simulink model "model"  (R2023b)
settings: Solver=VariableStepAuto  StartTime=0.0  StopTime=5  FixedStep=Tsi/10  RelTol=1e-4
undefined symbols (not defined in the file): B, B0, DiscIntNeverNeededParam, grtot, Hpp, Imax, In, Jm, Kdp_si, Ke, Ki_si, Kip_si, Kp_si, Kpp_si, Kppph_si, Kpppl_si, Kt, Kv, L, max_ppa_si, max_ppv_si, R, tauGp, Umax
libraries: simulink x10, slctrl_linear x1
(part 2 of 2)

== system model/EccB/current loop/current regulator ==
  current : Inport
  current_feedback : Inport  Port=2
  Scope : Scope  NumInputPorts=2
  Sum : Sum  Inputs=+-
  Sum2 : Sum
  Sum3 : Sum  Inputs=+-
  Sum4 : Sum  Inputs=++-
  Unit Delay : UnitDelay  SampleTime=-1  HasFrameUpgradeWarning=on
  integral gain : Gain  Gain=Ki_si*Tsi
  proportional gain : Gain  Gain=Kp_si
  voltage limitation : Saturate  UpperLimit=Umax  LowerLimit=-Umax
  voltage : Outport
  wires:
  voltage limitation/1 -> Scope/2, voltage/1, Sum3/2
  Sum3/1 -> Sum4/3
  Sum4/1 -> Unit Delay/1, Sum2/2  "ui(t)"
  Sum2/1 -> Sum3/1, Scope/1, voltage limitation/1  "u(t)"
  Sum/1 -> integral gain/1, proportional gain/1  "error"
  proportional gain/1 -> Sum2/1  "up(t)"
  current/1 -> Sum/1
  current_feedback/1 -> Sum/2
  Unit Delay/1 -> Sum4/1  "ui(t-1)"
  integral gain/1 -> Sum4/2

== system model/EccB/current loop/first order plant ==
  voltage : Inport
  Gain : Gain  Gain=1/tauM
  Gain5 : Gain  Gain=Kv
  Integrator : Integrator
  Integrator2 : Integrator
  Sum : Sum  Inputs=+-
  position : Outport
  velocity : Outport  Port=2
  wires:
  Integrator2/1 -> position/1
  voltage/1 -> Gain5/1
  Gain/1 -> Integrator/1
  Sum/1 -> Gain/1
  Integrator/1 -> Integrator2/1, velocity/1, Sum/2
  Gain5/1 -> Sum/1

== system model/EccB/current loop/power supply ==
  voltage setpoint : Inport
  Gain : Gain
  voltage : Outport
  wires:
  Gain/1 -> voltage/1
  voltage setpoint/1 -> Gain/1

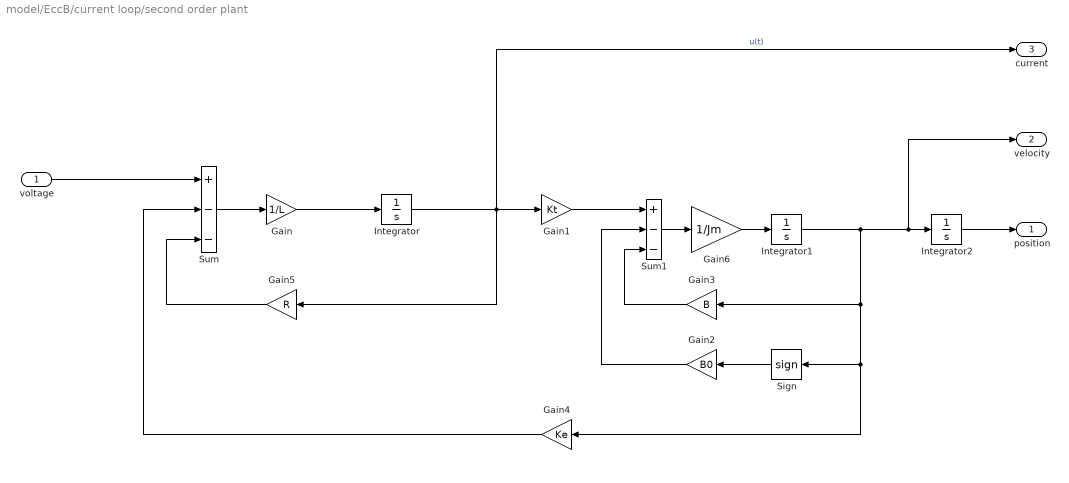
== system model/EccB/current loop/second order plant ==
  voltage : Inport
  Gain : Gain  Gain=1/L
  Gain1 : Gain  Gain=Kt
  Gain2 : Gain  Gain=B0
  Gain3 : Gain  Gain=B
  Gain4 : Gain  Gain=Ke
  Gain5 : Gain  Gain=R
  Gain6 : Gain  Gain=1/Jm
  Integrator : Integrator
  Integrator1 : Integrator
  Integrator2 : Integrator
  Sign : Signum
  Sum : Sum  Inputs=+--
  Sum1 : Sum  Inputs=+--
  position : Outport
  velocity : Outport  Port=2
  current : Outport  Port=3
  wires:
  Integrator2/1 -> position/1
  voltage/1 -> Sum/1
  Gain/1 -> Integrator/1
  Sum1/1 -> Gain6/1
  Gain5/1 -> Sum/3
  Gain6/1 -> Integrator1/1
  Gain4/1 -> Sum/2
  Sum/1 -> Gain/1
  Gain1/1 -> Sum1/1
  Sign/1 -> Gain2/1
  Gain3/1 -> Sum1/3
  Gain2/1 -> Sum1/2
  Integrator/1 -> current/1, Gain5/1, Gain1/1  "u(t)"
  Integrator1/1 -> velocity/1, Integrator2/1, Sign/1, Gain4/1, Gain3/1

== system model/EccB/path planner/devlta velocity ==
  Product : Product
  max acceleration : Constant  Value=max_ppa_si
  sampling time : Constant  Value=Tspp
  dw : Outport
  wires:
  sampling time/1 -> Product/1
  Product/1 -> dw/1
  max acceleration/1 -> Product/2

== system model/EccB/path planner/gain scheduler ==
  error : Inport
  Abs : Abs  SaturateOnIntegerOverflow=off
  Constant : Constant  Value=-Hpp
  Exp : Math
  Kp high : Constant  Value=Kppph_si
  Kp low : Constant  Value=Kpppl_si
  Product : Product
  Product1 : Product
  Sum : Sum  Inputs=+-
  Sum1 : Sum
  Km : Outport
  wires:
  Constant/1 -> Product/1
  Product/1 -> Exp/1
  Exp/1 -> Product1/1
  Abs/1 -> Product/2
  Kp low/1 -> Sum/1
  Kp high/1 -> Sum1/2, Sum/2
  Sum/1 -> Product1/2
  Product1/1 -> Sum1/1
  error/1 -> Abs/1
  Sum1/1 -> Km/1

== system model/EccB/path planner/setpoint correction ==
  speed : Inport
  feedback position : Inport  Port=2
  target position : Inport  Port=3
  AND : Logic  IconShape=distinctive  AllPortsSameDT=off  OutDataTypeStr=boolean
  AND1 : Logic  IconShape=distinctive  AllPortsSameDT=off  OutDataTypeStr=boolean
  Constant : Constant  Value=Active  OutDataTypeStr=boolean
  Constant2 : Constant  Value=0
  GreaterThan1 : RelationalOperator  Operator=>  OutDataTypeStr=boolean  RndMeth=Simplest  InputSameDT=off
  GreaterThan2 : RelationalOperator  Operator=<  OutDataTypeStr=boolean  RndMeth=Simplest  InputSameDT=off
  GreaterThan3 : RelationalOperator  Operator=<  OutDataTypeStr=boolean  RndMeth=Simplest  InputSameDT=off
  GreaterThan4 : RelationalOperator  Operator=>  OutDataTypeStr=boolean  RndMeth=Simplest  InputSameDT=off
  OR : Logic  Operator=OR  IconShape=distinctive  AllPortsSameDT=off  OutDataTypeStr=boolean
  Switch : Switch  Criteria=u2 > Threshold  SaturateOnIntegerOverflow=off  InputSameDT=off
  Terminator : Terminator
  motor velocity : Outport
  motor position : Outport  Port=2
  wires:
  GreaterThan3/1 -> AND1/1
  GreaterThan1/1 -> AND/2
  GreaterThan4/1 -> AND/1
  AND1/1 -> OR/2
  AND/1 -> OR/1
  Switch/1 -> motor position/1
  GreaterThan2/1 -> AND1/2
  speed/1 -> motor velocity/1  "filtered velocity"
  feedback position/1 -> GreaterThan2/2, Switch/1, GreaterThan1/2
  Constant2/1 -> GreaterThan3/2, GreaterThan4/2
  Constant/1 -> Switch/2
  OR/1 -> Terminator/1
  target position/1 -> Switch/3, GreaterThan3/1, GreaterThan2/1, GreaterThan1/1, GreaterThan4/1

== system model/EccB/position regulator/Integral + ant-windup ==
  error : Inport
  ui_old_sat : Inport  Port=2
  ui_old_no_sat : Inport  Port=3
  AND1 : Logic  IconShape=distinctive  AllPortsSameDT=off  OutDataTypeStr=boolean
  Constant1 : Constant  Value=0
  Ki : Gain  Gain=Kip_si*Tsp
  Relational Operator1 : RelationalOperator  Operator=~=  OutDataTypeStr=boolean  RndMeth=Simplest  InputSameDT=off
  Relational Operator3 : RelationalOperator  Operator=~=  OutDataTypeStr=boolean  RndMeth=Simplest  InputSameDT=off
  Sign1 : Signum
  Sign2 : Signum
  Sum1 : Sum
  Switch1 : Switch  Criteria=u2 > Threshold  SaturateOnIntegerOverflow=off  InputSameDT=off
  Unit Delay : UnitDelay  SampleTime=-1  HasFrameUpgradeWarning=on
  saturation : Saturate  UpperLimit=Imax  LowerLimit=-Imax
  ui (t) : Outport
  wires:
  Sign2/1 -> Relational Operator3/2
  error/1 -> Ki/1, Sign2/1
  Constant1/1 -> Switch1/1
  ui_old_sat/1 -> Relational Operator1/1
  ui_old_no_sat/1 -> Sign1/1, Relational Operator1/2
  Relational Operator3/1 -> AND1/2
  Relational Operator1/1 -> AND1/1
  Sign1/1 -> Relational Operator3/1
  AND1/1 -> Switch1/2
  Switch1/1 -> ui (t)/1, Unit Delay/1
  Sum1/1 -> saturation/1  "ui(t)"
  Ki/1 -> Sum1/1  "u(t)"
  Unit Delay/1 -> Sum1/2
  saturation/1 -> Switch1/3

== system model/LinB/current loop/current regulator ==
  current : Inport
  current_feedback : Inport  Port=2
  Scope : Scope  NumInputPorts=2
  Sum : Sum  Inputs=+-
  Sum2 : Sum
  Sum3 : Sum  Inputs=+-
  Sum4 : Sum  Inputs=++-
  Unit Delay : UnitDelay  SampleTime=-1  HasFrameUpgradeWarning=on
  integral gain : Gain  Gain=Ki_si*Tsi
  proportional gain : Gain  Gain=Kp_si
  voltage limitation : Saturate  UpperLimit=Umax  LowerLimit=-Umax
  voltage : Outport
  wires:
  voltage limitation/1 -> Scope/2, voltage/1, Sum3/2
  Sum3/1 -> Sum4/3
  Sum4/1 -> Unit Delay/1, Sum2/2  "ui(t)"
  Sum2/1 -> Sum3/1, Scope/1, voltage limitation/1  "u(t)"
  Sum/1 -> integral gain/1, proportional gain/1  "error"
  proportional gain/1 -> Sum2/1  "up(t)"
  current/1 -> Sum/1
  current_feedback/1 -> Sum/2
  Unit Delay/1 -> Sum4/1  "ui(t-1)"
  integral gain/1 -> Sum4/2

== system model/LinB/current loop/first order plant ==
  voltage : Inport
  Gain : Gain  Gain=1/tauM
  Gain5 : Gain  Gain=Kv
  Integrator : Integrator
  Integrator2 : Integrator
  Sum : Sum  Inputs=+-
  position : Outport
  velocity : Outport  Port=2
  wires:
  Integrator2/1 -> position/1
  voltage/1 -> Gain5/1
  Gain/1 -> Integrator/1
  Sum/1 -> Gain/1
  Integrator/1 -> Integrator2/1, velocity/1, Sum/2
  Gain5/1 -> Sum/1

== system model/LinB/current loop/power supply ==
  voltage setpoint : Inport
  Gain : Gain
  voltage : Outport
  wires:
  Gain/1 -> voltage/1
  voltage setpoint/1 -> Gain/1

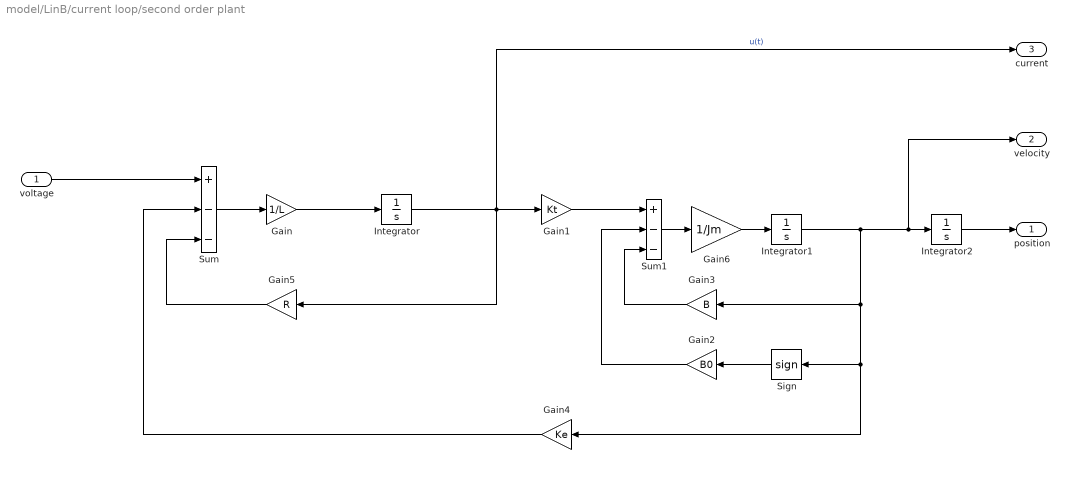
== system model/LinB/current loop/second order plant ==
  voltage : Inport
  Gain : Gain  Gain=1/L
  Gain1 : Gain  Gain=Kt
  Gain2 : Gain  Gain=B0
  Gain3 : Gain  Gain=B
  Gain4 : Gain  Gain=Ke
  Gain5 : Gain  Gain=R
  Gain6 : Gain  Gain=1/Jm
  Integrator : Integrator
  Integrator1 : Integrator
  Integrator2 : Integrator
  Sign : Signum
  Sum : Sum  Inputs=+--
  Sum1 : Sum  Inputs=+--
  position : Outport
  velocity : Outport  Port=2
  current : Outport  Port=3
  wires:
  Integrator2/1 -> position/1
  voltage/1 -> Sum/1
  Gain/1 -> Integrator/1
  Sum1/1 -> Gain6/1
  Gain5/1 -> Sum/3
  Gain6/1 -> Integrator1/1
  Gain4/1 -> Sum/2
  Sum/1 -> Gain/1
  Gain1/1 -> Sum1/1
  Sign/1 -> Gain2/1
  Gain3/1 -> Sum1/3
  Gain2/1 -> Sum1/2
  Integrator/1 -> current/1, Gain5/1, Gain1/1  "u(t)"
  Integrator1/1 -> velocity/1, Integrator2/1, Sign/1, Gain4/1, Gain3/1

== system model/LinB/path planner/devlta velocity ==
  Product : Product
  max acceleration : Constant  Value=max_ppa_si
  sampling time : Constant  Value=Tspp
  dw : Outport
  wires:
  sampling time/1 -> Product/1
  Product/1 -> dw/1
  max acceleration/1 -> Product/2

== system model/LinB/path planner/gain scheduler ==
  error : Inport
  Abs : Abs  SaturateOnIntegerOverflow=off
  Constant : Constant  Value=-Hpp
  Exp : Math
  Kp high : Constant  Value=Kppph_si
  Kp low : Constant  Value=Kpppl_si
  Product : Product
  Product1 : Product
  Sum : Sum  Inputs=+-
  Sum1 : Sum
  Km : Outport
  wires:
  Constant/1 -> Product/1
  Product/1 -> Exp/1
  Exp/1 -> Product1/1
  Abs/1 -> Product/2
  Kp low/1 -> Sum/1
  Kp high/1 -> Sum1/2, Sum/2
  Sum/1 -> Product1/2
  Product1/1 -> Sum1/1
  error/1 -> Abs/1
  Sum1/1 -> Km/1

== system model/LinB/path planner/setpoint correction ==
  speed : Inport
  feedback position : Inport  Port=2
  target position : Inport  Port=3
  AND : Logic  IconShape=distinctive  AllPortsSameDT=off  OutDataTypeStr=boolean
  AND1 : Logic  IconShape=distinctive  AllPortsSameDT=off  OutDataTypeStr=boolean
  Constant : Constant  Value=Active  OutDataTypeStr=boolean
  Constant2 : Constant  Value=0
  GreaterThan1 : RelationalOperator  Operator=>  OutDataTypeStr=boolean  RndMeth=Simplest  InputSameDT=off
  GreaterThan2 : RelationalOperator  Operator=<  OutDataTypeStr=boolean  RndMeth=Simplest  InputSameDT=off
  GreaterThan3 : RelationalOperator  Operator=<  OutDataTypeStr=boolean  RndMeth=Simplest  InputSameDT=off
  GreaterThan4 : RelationalOperator  Operator=>  OutDataTypeStr=boolean  RndMeth=Simplest  InputSameDT=off
  OR : Logic  Operator=OR  IconShape=distinctive  AllPortsSameDT=off  OutDataTypeStr=boolean
  Switch : Switch  Criteria=u2 > Threshold  SaturateOnIntegerOverflow=off  InputSameDT=off
  Terminator : Terminator
  motor velocity : Outport
  motor position : Outport  Port=2
  wires:
  GreaterThan3/1 -> AND1/1
  GreaterThan1/1 -> AND/2
  GreaterThan4/1 -> AND/1
  AND1/1 -> OR/2
  AND/1 -> OR/1
  Switch/1 -> motor position/1
  GreaterThan2/1 -> AND1/2
  speed/1 -> motor velocity/1  "filtered velocity"
  feedback position/1 -> GreaterThan2/2, Switch/1, GreaterThan1/2
  Constant2/1 -> GreaterThan3/2, GreaterThan4/2
  Constant/1 -> Switch/2
  OR/1 -> Terminator/1
  target position/1 -> Switch/3, GreaterThan3/1, GreaterThan2/1, GreaterThan1/1, GreaterThan4/1

== system model/LinB/position regulator/Integral + ant-windup ==
  error : Inport
  ui_old_sat : Inport  Port=2
  ui_old_no_sat : Inport  Port=3
  AND1 : Logic  IconShape=distinctive  AllPortsSameDT=off  OutDataTypeStr=boolean
  Constant1 : Constant  Value=0
  Ki : Gain  Gain=Kip_si*Tsp
  Relational Operator1 : RelationalOperator  Operator=~=  OutDataTypeStr=boolean  RndMeth=Simplest  InputSameDT=off
  Relational Operator3 : RelationalOperator  Operator=~=  OutDataTypeStr=boolean  RndMeth=Simplest  InputSameDT=off
  Sign1 : Signum
  Sign2 : Signum
  Sum1 : Sum
  Switch1 : Switch  Criteria=u2 > Threshold  SaturateOnIntegerOverflow=off  InputSameDT=off
  Unit Delay : UnitDelay  SampleTime=-1  HasFrameUpgradeWarning=on
  saturation : Saturate  UpperLimit=In  LowerLimit=-In
  ui (t) : Outport
  wires:
  Sign2/1 -> Relational Operator3/2
  error/1 -> Ki/1, Sign2/1
  Constant1/1 -> Switch1/1
  ui_old_sat/1 -> Relational Operator1/1
  ui_old_no_sat/1 -> Sign1/1, Relational Operator1/2
  Relational Operator3/1 -> AND1/2
  Relational Operator1/1 -> AND1/1
  Sign1/1 -> Relational Operator3/1
  AND1/1 -> Switch1/2
  Switch1/1 -> ui (t)/1, Unit Delay/1
  Sum1/1 -> saturation/1  "ui(t)"
  Ki/1 -> Sum1/1  "u(t)"
  Unit Delay/1 -> Sum1/2
  saturation/1 -> Switch1/3

== system model/Test Actuator/current loop/current regulator ==
  current : Inport
  current_feedback : Inport  Port=2
  Scope : Scope  NumInputPorts=2
  Sum : Sum  Inputs=+-
  Sum2 : Sum
  Sum3 : Sum  Inputs=+-
  Sum4 : Sum  Inputs=++-
  Unit Delay : UnitDelay  SampleTime=-1  HasFrameUpgradeWarning=on
  integral gain : Gain  Gain=Ki_si*Tsi
  proportional gain : Gain  Gain=Kp_si
  voltage limitation : Saturate  UpperLimit=Umax  LowerLimit=-Umax
  voltage : Outport
  wires:
  voltage limitation/1 -> Scope/2, voltage/1, Sum3/2
  Sum3/1 -> Sum4/3
  Sum4/1 -> Unit Delay/1, Sum2/2  "ui(t)"
  Sum2/1 -> Sum3/1, Scope/1, voltage limitation/1  "u(t)"
  Sum/1 -> integral gain/1, proportional gain/1  "error"
  proportional gain/1 -> Sum2/1  "up(t)"
  current/1 -> Sum/1
  current_feedback/1 -> Sum/2
  Unit Delay/1 -> Sum4/1  "ui(t-1)"
  integral gain/1 -> Sum4/2

== system model/Test Actuator/current loop/first order plant ==
  voltage : Inport
  Gain : Gain  Gain=1/tauM
  Gain5 : Gain  Gain=Kv
  Integrator : Integrator
  Integrator2 : Integrator
  Sum : Sum  Inputs=+-
  position : Outport
  velocity : Outport  Port=2
  wires:
  Integrator2/1 -> position/1
  voltage/1 -> Gain5/1
  Gain/1 -> Integrator/1
  Sum/1 -> Gain/1
  Integrator/1 -> Integrator2/1, velocity/1, Sum/2
  Gain5/1 -> Sum/1

== system model/Test Actuator/current loop/power supply ==
  voltage setpoint : Inport
  Gain : Gain
  voltage : Outport
  wires:
  Gain/1 -> voltage/1
  voltage setpoint/1 -> Gain/1

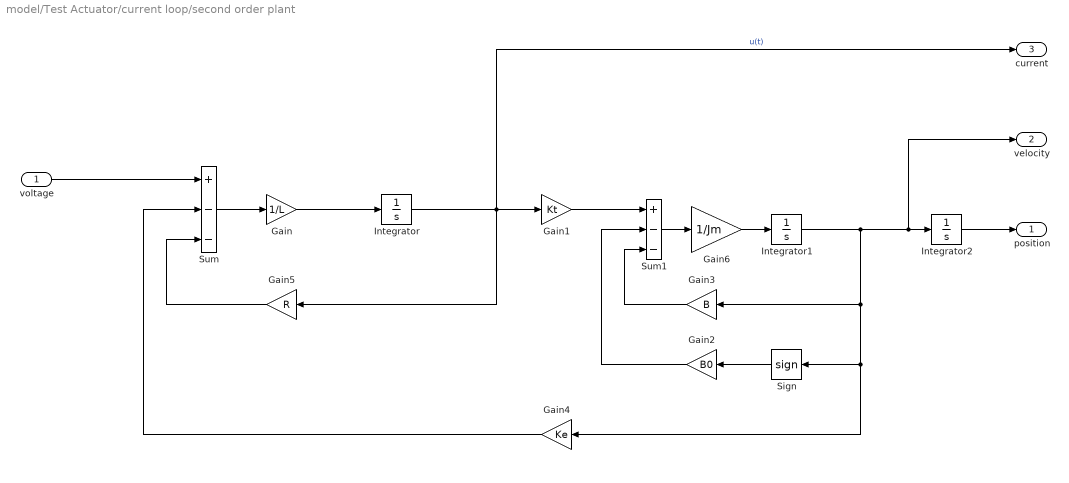
== system model/Test Actuator/current loop/second order plant ==
  voltage : Inport
  Gain : Gain  Gain=1/L
  Gain1 : Gain  Gain=Kt
  Gain2 : Gain  Gain=B0
  Gain3 : Gain  Gain=B
  Gain4 : Gain  Gain=Ke
  Gain5 : Gain  Gain=R
  Gain6 : Gain  Gain=1/Jm
  Integrator : Integrator
  Integrator1 : Integrator
  Integrator2 : Integrator
  Sign : Signum
  Sum : Sum  Inputs=+--
  Sum1 : Sum  Inputs=+--
  position : Outport
  velocity : Outport  Port=2
  current : Outport  Port=3
  wires:
  Integrator2/1 -> position/1
  voltage/1 -> Sum/1
  Gain/1 -> Integrator/1
  Sum1/1 -> Gain6/1
  Gain5/1 -> Sum/3
  Gain6/1 -> Integrator1/1
  Gain4/1 -> Sum/2
  Sum/1 -> Gain/1
  Gain1/1 -> Sum1/1
  Sign/1 -> Gain2/1
  Gain3/1 -> Sum1/3
  Gain2/1 -> Sum1/2
  Integrator/1 -> current/1, Gain5/1, Gain1/1  "u(t)"
  Integrator1/1 -> velocity/1, Integrator2/1, Sign/1, Gain4/1, Gain3/1

== system model/Test Actuator/path planner/devlta velocity ==
  Product : Product
  max acceleration : Constant  Value=max_ppa_si
  sampling time : Constant  Value=Tspp
  dw : Outport
  wires:
  sampling time/1 -> Product/1
  Product/1 -> dw/1
  max acceleration/1 -> Product/2

== system model/Test Actuator/path planner/gain scheduler ==
  error : Inport
  Abs : Abs  SaturateOnIntegerOverflow=off
  Constant : Constant  Value=-Hpp
  Exp : Math
  Kp high : Constant  Value=Kppph_si
  Kp low : Constant  Value=Kpppl_si
  Product : Product
  Product1 : Product
  Sum : Sum  Inputs=+-
  Sum1 : Sum
  Km : Outport
  wires:
  Constant/1 -> Product/1
  Product/1 -> Exp/1
  Exp/1 -> Product1/1
  Abs/1 -> Product/2
  Kp low/1 -> Sum/1
  Kp high/1 -> Sum1/2, Sum/2
  Sum/1 -> Product1/2
  Product1/1 -> Sum1/1
  error/1 -> Abs/1
  Sum1/1 -> Km/1

== system model/Test Actuator/path planner/setpoint correction ==
  speed : Inport
  feedback position : Inport  Port=2
  target position : Inport  Port=3
  AND : Logic  IconShape=distinctive  AllPortsSameDT=off  OutDataTypeStr=boolean
  AND1 : Logic  IconShape=distinctive  AllPortsSameDT=off  OutDataTypeStr=boolean
  Constant : Constant  Value=Active  OutDataTypeStr=boolean
  Constant2 : Constant  Value=0
  GreaterThan1 : RelationalOperator  Operator=>  OutDataTypeStr=boolean  RndMeth=Simplest  InputSameDT=off
  GreaterThan2 : RelationalOperator  Operator=<  OutDataTypeStr=boolean  RndMeth=Simplest  InputSameDT=off
  GreaterThan3 : RelationalOperator  Operator=<  OutDataTypeStr=boolean  RndMeth=Simplest  InputSameDT=off
  GreaterThan4 : RelationalOperator  Operator=>  OutDataTypeStr=boolean  RndMeth=Simplest  InputSameDT=off
  OR : Logic  Operator=OR  IconShape=distinctive  AllPortsSameDT=off  OutDataTypeStr=boolean
  Switch : Switch  Criteria=u2 > Threshold  SaturateOnIntegerOverflow=off  InputSameDT=off
  Terminator : Terminator
  motor velocity : Outport
  motor position : Outport  Port=2
  wires:
  GreaterThan3/1 -> AND1/1
  GreaterThan1/1 -> AND/2
  GreaterThan4/1 -> AND/1
  AND1/1 -> OR/2
  AND/1 -> OR/1
  Switch/1 -> motor position/1
  GreaterThan2/1 -> AND1/2
  speed/1 -> motor velocity/1  "filtered velocity"
  feedback position/1 -> GreaterThan2/2, Switch/1, GreaterThan1/2
  Constant2/1 -> GreaterThan3/2, GreaterThan4/2
  Constant/1 -> Switch/2
  OR/1 -> Terminator/1
  target position/1 -> Switch/3, GreaterThan3/1, GreaterThan2/1, GreaterThan1/1, GreaterThan4/1

== system model/Test Actuator/position regulator/Integral + ant-windup ==
  error : Inport
  ui_old_sat : Inport  Port=2
  ui_old_no_sat : Inport  Port=3
  AND1 : Logic  IconShape=distinctive  AllPortsSameDT=off  OutDataTypeStr=boolean
  Constant1 : Constant  Value=0
  Ki : Gain  Gain=Kip_si*Tsp
  Relational Operator1 : RelationalOperator  Operator=~=  OutDataTypeStr=boolean  RndMeth=Simplest  InputSameDT=off
  Relational Operator3 : RelationalOperator  Operator=~=  OutDataTypeStr=boolean  RndMeth=Simplest  InputSameDT=off
  Sign1 : Signum
  Sign2 : Signum
  Sum1 : Sum
  Switch1 : Switch  Criteria=u2 > Threshold  SaturateOnIntegerOverflow=off  InputSameDT=off
  Unit Delay : UnitDelay  SampleTime=-1  HasFrameUpgradeWarning=on
  saturation : Saturate  UpperLimit=In  LowerLimit=-In
  ui (t) : Outport
  wires:
  Sign2/1 -> Relational Operator3/2
  error/1 -> Ki/1, Sign2/1
  Constant1/1 -> Switch1/1
  ui_old_sat/1 -> Relational Operator1/1
  ui_old_no_sat/1 -> Sign1/1, Relational Operator1/2
  Relational Operator3/1 -> AND1/2
  Relational Operator1/1 -> AND1/1
  Sign1/1 -> Relational Operator3/1
  AND1/1 -> Switch1/2
  Switch1/1 -> ui (t)/1, Unit Delay/1
  Sum1/1 -> saturation/1  "ui(t)"
  Ki/1 -> Sum1/1  "u(t)"
  Unit Delay/1 -> Sum1/2
  saturation/1 -> Switch1/3

== matlab function model/MATLAB Function ==
  data: acceleration output; velocity output; target_position input; delay input; target_position output; feedback_position input; Tspp parameter; max_ppa_si parameter; max_ppv_si parameter; Kppph_si parameter; Kpppl_si parameter; Hpp parameter; velocity_offset parameter; synch_to_target_ratio parameter
function [acceleration, velocity, target_position] = path_planner(target_position, delay, feedback_position, ...
                                                                  Tspp, ... %mask parameters (no function inputs)
                                                                  max_ppa_si, ...
                                                                  max_ppv_si, ...
                                                                  Kppph_si, ...
                                                                  Kpppl_si, ...
                                                                  Hpp, ...
                                                                  velocity_offset, ...
                                                                  synch_to_target_ratio) ...

    % save position, velocity and acceleration old values
    persistent position_old;
    persistent velocity_old;
    persistent acceleration_old; %#ok<PUSE>
    if isempty(position_old)
        position_old = 0;
        velocity_old = 0;
        acceleration_old = 0; %#ok<NASGU> 
    end

    % Current position error (target vs feedback). The selected feedback
    % should be always the one of the actuator with the slowest dynamics,
    % in this case EccB. In this way the path planner adaptive control
    % action is limited by it (this avoids big oscillations). In case
    % another actuator is the slowest one, and it is a linear one, we need
    % also the linear to angular map for EccB.
    error = target_position - feedback_position;

    % run gain scheduler (adaptive control)
    Km = gain_scheduler(error);

    % raw velocity (path planner system input)
    velocity = error*Km;

    % Synchronization correction, it always opposes to the steering force,
    % in case the commanded velocity is zero (the slow actuator reached the
    % target), don't apply the correction, the other actuators will
    % recover quickly and reduce the gap.
    if velocity > velocity_offset
        velocity = velocity - synch_to_target_ratio*Km*delay;
    elseif velocity < -velocity_offset
        velocity = velocity + synch_to_target_ratio*Km*delay;
    end

    % get runtime velocity boundaries (consider max acceleration)
    velocity_high = min(velocity_old + max_ppa_si*Tspp, max_ppv_si);
    velocity_low = max(velocity_old - max_ppa_si*Tspp, -max_ppv_si);
    velocity = min(max(velocity, velocity_low), velocity_high);

    % Forward kinematics simulation for position (speed integral). Also the
    % real position feedback of the slowest actuator could be used in order
    % to increase the reactivity of the path planner, however this
    % introduces oscillations and jumps in the commanded velocity that
    % consequently cause oscillations on the actual position and so on.
    target_position = position_old + Tspp*velocity;

    % real requested acceleration (can also be removed if not used)
    acceleration = (velocity - velocity_old)/Tspp;

    % save position, velocity and acceleration (for next cycle)
    position_old = target_position;
    velocity_old = velocity;
    acceleration_old = acceleration;

    function gain = gain_scheduler(error)
    %
    % Compute optimal proportional gain according to position error.
    %
        gain = Kppph_si + (Kpppl_si - Kppph_si)*(1 / (1 + Hpp*abs(error)));
    end

end

== matlab function model/angular-linear-map ==
  data: x input; x output
function x = deg2m_r(x)
%
% EccA-EccB angular [deg] to linear [m] motion map for rear axis.
%
    c5 = 0.0000000000624;
    c4 = -0.000000000045;
    c3 = -0.0000037025199;
    c2 = -0.0001050951019;
    c1 = 0.0716813513211;
    c0 = 0.0041785649983;
    x = 0.001*(c5*x.^5 + c4*x.^4 + c3*x.^3 + c2*x.^2 + c1*x + c0);
end

== matlab function model/map ==
  data: x input; x output
function x = deg2m_r(x)
%
% EccA-EccB angular [deg] to linear [m] motion map for rear axis.
%
    c5 = 0.0000000000624;
    c4 = -0.000000000045;
    c3 = -0.0000037025199;
    c2 = -0.0001050951019;
    c1 = 0.0716813513211;
    c0 = 0.0041785649983;
    x = 0.001*(c5*x.^5 + c4*x.^4 + c3*x.^3 + c2*x.^2 + c1*x + c0);
end

== matlab function model/map1 ==
  data: x input; x output
function x = deg2m_r(x)
%
% EccA-EccB angular [deg] to linear [m] motion map for rear axis.
%
    c5 = 0.0000000000624;
    c4 = -0.000000000045;
    c3 = -0.0000037025199;
    c2 = -0.0001050951019;
    c1 = 0.0716813513211;
    c0 = 0.0041785649983;
    x = 0.001*(c5*x.^5 + c4*x.^4 + c3*x.^3 + c2*x.^2 + c1*x + c0);
end

== matlab function model/angular-linear-map2 ==
  data: x input; x output
function x = deg2m_r(x)
%
% EccA-EccB angular [deg] to linear [m] motion map for rear axis.
%
    c5 = 0.0000000000624;
    c4 = -0.000000000045;
    c3 = -0.0000037025199;
    c2 = -0.0001050951019;
    c1 = 0.0716813513211;
    c0 = 0.0041785649983;
    x = 0.001*(c5*x.^5 + c4*x.^4 + c3*x.^3 + c2*x.^2 + c1*x + c0);
end
